simulink model "VehicleModel"  (R2020b)
settings: Solver=FixedStepAuto  StartTime=0.0  StopTime=1068  FixedStep=0.1  RelTol=1e-3
model workspace (MAT data in the model file):
  t : mpt.Parameter (value not decoded)
(part 4 of 5)

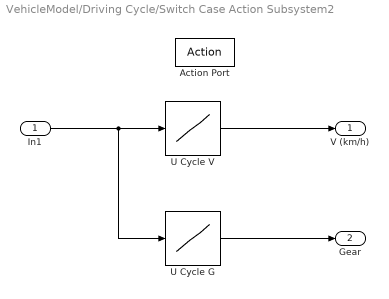
== system VehicleModel/Driving Cycle/Switch Case Action Subsystem2 ==
  In1 : Inport
  Action Port : ActionPort  ActionPortLabel=case [ 2 ]:
  " U Cycle V" : Lookup_n-D  NumberOfTableDimensions=1  BreakpointsForDimension1=|  Table=|  InternalRulePriority=Speed  RndMeth=Simplest  InputSameDT=on
      | [0
      | 1
      | 2
      | 3
      | 4
      | 5
      | 6
      | 7
      | 8
      | 9
      | 10
      | 11
      | 12
      | 13
      | 14
      | 15
      | 16
      | 17
      | 18
      | 19
      | 20
      | 21
      | 22
      | 23
      | 24
      | 25
      | 26
      | 27
      | 28
      | 29
      | 30
      | 31
      | 32
      | 33
      | 34
      | 35
      | 36
      | 37
      | 38
      | 39
      | 40
      | 41
      | 42
      | 43
      | 44
      | 45
      | 46
      | 47
      | 48
      | 49
      | 50
      | 51
      | 52
      | 53
      | 54
      | 55
      | 56
      | 57
      | 58
      | 59
      | 60
      | 61
      | 62
      | 63
      | 64
      | 65
      | 66
      | 67
      | 68
      | 69
      | 70
      | 71
      | 72
      | 73
      | 74
      | 75
      | 76
      | 77
      | 78
      | 79
      | 80
      | 81
      | 82
      | 83
      | 84
      | 85
      | 86
      | 87
      | 88
      | 89
      | 90
      | 91
      | 92
      | 93
      | 94
      | 95
      | 96
      | 97
      | 98
      | 99
      | 100
      | 101
      | 102
      | 103
      | 104
      | 105
      | 106
      | 107
      | 108
      | 109
      | 110
      | 111
      | 112
      | 113
      | 114
      | 115
      | 116
      | 117
      | 118
      | 119
      | 120
      | 121
      | 122
      | 123
      | 124
      | 125
      | 126
      | 127
      | 128
      | 129
      | 130
      | 131
      | 132
      | 133
      | 134
      | 135
      | 136
      | 137
      | 138
      | 139
      | 140
      | 141
      | 142
      | 143
      | 144
      | 145
      | 146
      | 147
      | 148
      | 149
      | 150
      | 151
      | 152
      | 153
      | 154
      | 155
      | 156
      | 157
      | 158
      | 159
      | 160
      | 161
      | 162
      | 163
      | 164
      | 165
      | 166
      | 167
      | 168
      | 169
      | 170
      | 171
      | 172
      | 173
      | 174
      | 175
      | 176
      | 177
      | 178
      | 179
      | 180
      | 181
      | 182
      | 183
      | 184
      | 185
      | 186
      | 187
      | 188
      | 189
      | 190
      | 191
      | 192
      | 193
      | 194
      | 195
      | 196
      | 197
      | 198
      | 199
      | 200
      | 201
      | 202
      | 203
      | 204
      | 205
      | 206
      | 207
      | 208
      | 209
      | 210
      | 211
      | 212
      | 213
      | 214
      | 215
      | 216
      | 217
      | 218
      | 219
      | 220
      | 221
      | 222
      | 223
      | 224
      | 225
      | 226
      | 227
      | 228
      | 229
      | 230
      | 231
      | 232
      | 233
      | 234
      | 235
      | 236
      | 237
      | 238
      | 239
      | 240
      | 241
      | 242
      | 243
      | 244
      | 245
      | 246
      | 247
      | 248
      | 249
      | 250
      | 251
      | 252
      | 253
      | 254
      | 255
      | 256
      | 257
      | 258
      | 259
      | 260
      | 261
      | 262
      | 263
      | 264
      | 265
      | 266
      | 267
      | 268
      | 269
      | 270
      | 271
      | 272
      | 273
      | 274
      | 275
      | 276
      | 277
      | 278
      | 279
      | 280
      | 281
      | 282
      | 283
      | 284
      | 285
      | 286
      | 287
      | 288
      | 289
      | 290
      | 291
      | 292
      | 293
      | 294
      | 295
      | 296
      | 297
      | 298
      | 299
      | 300
      | 301
      | 302
      | 303
      | 304
      | 305
      | 306
      | 307
      | 308
      | 309
      | 310
      | 311
      | 312
      | 313
      | 314
      | 315
      | 316
      | 317
      | 318
      | 319
      | 320
      | 321
      | 322
      | 323
      | 324
      | 325
      | 326
      | 327
      | 328
      | 329
      | 330
      | 331
      | 332
      | 333
      | 334
      | 335
      | 336
      | 337
      | 338
      | 339
      | 340
      | 341
      | 342
      | 343
      | 344
      | 345
      | 346
      | 347
      | 348
      | 349
      | 350
      | 351
      | 352
      | 353
      | 354
      | 355
      | 356
      | 357
      | 358
      | 359
      | 360
      | 361
      | 362
      | 363
      | 364
      | 365
      | 366
      | 367
      | 368
      | 369
      | 370
      | 371
      | 372
      | 373
      | 374
      | 375
      | 376
      | 377
      | 378
      | 379
      | 380
      | 381
      | 382
      | 383
      | 384
      | 385
      | 386
      | 387
      | 388
      | 389
      | 390
      | 391
      | 392
      | 393
      | 394
      | 395
      | 396
      | 397
      | 398
      | 399
      | 400
      | 401
      | 402
      | 403
      | 404
      | 405
      | 406
      | 407
      | 408
      | 409
      | 410
      | 411
      | 412
      | 413
      | 414
      | 415
      | 416
      | 417
      | 418
      | 419
      | 420
      | 421
      | 422
      | 423
      | 424
      | 425
      | 426
      | 427
      | 428
      | 429
      | 430
      | 431
      | 432
      | 433
      | 434
      | 435
      | 436
      | 437
      | 438
      | 439
      | 440
      | 441
      | 442
      | 443
      | 444
      | 445
      | 446
      | 447
      | 448
      | 449
      | 450
      | 451
      | 452
      | 453
      | 454
      | 455
      | 456
      | 457
      | 458
      | 459
      | 460
      | 461
      | 462
      | 463
      | 464
      | 465
      | 466
      | 467
      | 468
      | 469
      | 470
      | 471
      | 472
      | 473
      | 474
      | 475
      | 476
      | 477
      | 478
      | 479
      | 480
      | 481
      | 482
      | 483
      | 484
      | 485
      | 486
      | 487
      | 488
      | 489
      | 490
      | 491
      | 492
      | 493
      | 494
      | 495
      | 496
      | 497
      | 498
      | 499
      | 500
      | 501
      | 502
      | 503
      | 504
      | 505
      | 506
      | 507
      | 508
      | 509
      | 510
      | 511
      | 512
      | 513
      | 514
      | 515
      | 516
      | 517
      | 518
      | 519
      | 520
      | 521
      | 522
      | 523
      | 524
      | 525
      | 526
      | 527
      | 528
      | 529
      | 530
      | 531
      | 532
      | 533
      | 534
      | 535
      | 536
      | 537
      | 538
      | 539
      | 540
      | 541
      | 542
      | 543
      | 544
      | 545
      | 546
      | 547
      | 548
      | 549
      | 550
      | 551
      | 552
      | 553
      | 554
      | 555
      | 556
      | 557
      | 558
      | 559
      | 560
      | 561
      | 562
      | 563
      | 564
      | 565
      | 566
      | 567
      | 568
      | 569
      | 570
      | 571
      | 572
      | 573
      | 574
      | 575
      | 576
      | 577
      | 578
      | 579
      | 580
      | 581
      | 582
      | 583
      | 584
      | 585
      | 586
      | 587
      | 588
      | 589
      | 590
      | 591
      | 592
      | 593
      | 594
      | 595
      | 596
      | 597
      | 598
      | 599
      | 600
      | 601
      | 602
      | 603
      | 604
      | 605
      | 606
      | 607
      | 608
      | 609
      | 610
      | 611
      | 612
      | 613
      | 614
      | 615
      | 616
      | 617
      | 618
      | 619
      | 620
      | 621
      | 622
      | 623
      | 624
      | 625
      | 626
      | 627
      | 628
      | 629
      | 630
      | 631
      | 632
      | 633
      | 634
      | 635
      | 636
      | 637
      | 638
      | 639
      | 640
      | 641
      | 642
      | 643
      | 644
      | 645
      | 646
      | 647
      | 648
      | 649
      | 650
      | 651
      | 652
      | 653
      | 654
      | 655
      | 656
      | 657
      | 658
      | 659
      | 660
      | 661
      | 662
      | 663
      | 664
      | 665
      | 666
      | 667
      | 668
      | 669
      | 670
      | 671
      | 672
      | 673
      | 674
      | 675
      | 676
      | 677
      | 678
      | 679
      | 680
      | 681
      | 682
      | 683
      | 684
      | 685
      | 686
      | 687
      | 688
      | 689
      | 690
      | 691
      | 692
      | 693
      | 694
      | 695
      | 696
      | 697
      | 698
      | 699
      | 700
      | 701
      | 702
      | 703
      | 704
      | 705
      | 706
      | 707
      | 708
      | 709
      | 710
      | 711
      | 712
      | 713
      | 714
      | 715
      | 716
      | 717
      | 718
      | 719
      | 720
      | 721
      | 722
      | 723
      | 724
      | 725
      | 726
      | 727
      | 728
      | 729
      | 730
      | 731
      | 732
      | 733
      | 734
      | 735
      | 736
      | 737
      | 738
      | 739
      | 740
      | 741
      | 742
      | 743
      | 744
      | 745
      | 746
      | 747
      | 748
      | 749
      | 750
      | 751
      | 752
      | 753
      | 754
      | 755
      | 756
      | 757
      | 758
      | 759
      | 760
      | 761
      | 762
      | 763
      | 764
      | 765
      | 766
      | 767
      | 768
      | 769
      | 770
      | 771
      | 772
      | 773
      | 774
      | 775
      | 776
      | 777
      | 778
      | 779
      | 780
      | 781
      | 782
      | 783
      | 784
      | 785
      | 786
      | 787
      | 788
      | 789
      | 790
      | 791
      | 792
      | 793
      | 794
      | 795
      | 796
      | 797
      | 798
      | 799
      | 800
      | 801
      | 802
      | 803
      | 804
      | 805
      | 806
      | 807
      | 808
      | 809
      | 810
      | 811
      | 812
      | 813
      | 814
      | 815
      | 816
      | 817
      | 818
      | 819
      | 820
      | 821
      | 822
      | 823
      | 824
      | 825
      | 826
      | 827
      | 828
      | 829
      | 830
      | 831
      | 832
      | 833
      | 834
      | 835
      | 836
      | 837
      | 838
      | 839
      | 840
      | 841
      | 842
      | 843
      | 844
      | 845
      | 846
      | 847
      | 848
      | 849
      | 850
      | 851
      | 852
      | 853
      | 854
      | 855
      | 856
      | 857
      | 858
      | 859
      | 860
      | 861
      | 862
      | 863
      | 864
      | 865
      | 866
      | 867
      | 868
      | 869
      | 870
      | 871
      | 872
      | 873
      | 874
      | 875
      | 876
      | 877
      | 878
      | 879
      | 880
      | 881
      | 882
      | 883
      | 884
      | 885
      | 886
      | 887
      | 888
      | 889
      | 890
      | 891
      | 892
      | 893
      | 894
      | 895
      | 896
      | 897
      | 898
      | 899
      | 900
      | 901
      | 902
      | 903
      | 904
      | 905
      | 906
      | 907
      | 908
      | 909
      | 910
      | 911
      | 912
      | 913
      | 914
      | 915
      | 916
      | 917
      | 918
      | 919
      | 920
      | 921
      | 922
      | 923
      | 924
      | 925
      | 926
      | 927
      | 928
      | 929
      | 930
      | 931
      | 932
      | 933
      | 934
      | 935
      | 936
      | 937
      | 938
      | 939
      | 940
      | 941
      | 942
      | 943
      | 944
      | 945
      | 946
      | 947
      | 948
      | 949
      | 950
      | 951
      | 952
      | 953
      | 954
      | 955
      | 956
      | 957
      | 958
      | 959
      | 960
      | 961
      | 962
      | 963
      | 964
      | 965
      | 966
      | 967
      | 968
      | 969
      | 970
      | 971
      | 972
      | 973
      | 974
      | 975
      | 976
      | 977
      | 978
      | 979
      | 980
      | 981
      | 982
      | 983
      | 984
      | 985
      | 986
      | 987
      | 988
      | 989
      | 990
      | 991
      | 992
      | 993]
      | [0
      | 0
      | 0
      | 0
      | 0
      | 0
      | 0
      | 0
      | 0
      | 0
      | 0
      | 0
      | 0
      | 0
      | 0
      | 0
      | 0
      | 0
      | 0
      | 0
      | 0
      | 0.700000000000000
      | 2.10000000000000
      | 9.20000000000000
      | 15.6000000000000
      | 19.8000000000000
      | 19.8000000000000
      | 22.7000000000000
      | 25.5000000000000
      | 29.8000000000000
      | 34
      | 36.9000000000000
      | 38.3000000000000
      | 40.4000000000000
      | 43.2000000000000
      | 46.1000000000000
      | 46.1000000000000
      | 46.1000000000000
      | 44.6000000000000
      | 46.1000000000000
      | 48.2000000000000
      | 48.9000000000000
      | 48.2000000000000
      | 46.8000000000000
      | 44.6000000000000
      | 42.5000000000000
      | 41.8000000000000
      | 41.1000000000000
      | 39.7000000000000
      | 36.1000000000000
      | 34.7000000000000
      | 34.7000000000000
      | 36.9000000000000
      | 36.1000000000000
      | 36.1000000000000
      | 34.7000000000000
      | 32.6000000000000
      | 29.1000000000000
      | 24.1000000000000
      | 20.6000000000000
      | 15.6000000000000
      | 11.3000000000000
      | 9.20000000000000
      | 9.20000000000000
      | 9.20000000000000
      | 9.90000000000000
      | 10.6000000000000
      | 12
      | 11.3000000000000
      | 7.80000000000000
      | 1.40000000000000
      | 0
      | 0
      | 0
      | 0
      | 0
      | 0
      | 0
      | 0
      | 0
      | 0
      | 0
      | 0
      | 0
      | 0
      | 0
      | 0
      | 0
      | 0
      | 0
      | 0
      | 0
      | 0
      | 0.700000000000000
      | 2.10000000000000
      | 9.20000000000000
      | 15.6000000000000
      | 19.8000000000000
      | 19.8000000000000
      | 22.7000000000000
      | 25.5000000000000
      | 29.8000000000000
      | 34
      | 36.9000000000000
      | 38.3000000000000
      | 40.4000000000000
      | 43.2000000000000
      | 46.1000000000000
      | 46.1000000000000
      | 46.1000000000000
      | 44.6000000000000
      | 46.1000000000000
      | 48.2000000000000
      | 48.9000000000000
      | 48.2000000000000
      | 46.8000000000000
      | 44.6000000000000
      | 42.5000000000000
      | 41.8000000000000
      | 41.1000000000000
      | 39.7000000000000
      | 36.1000000000000
      | 34.7000000000000
      | 34.7000000000000
      | 36.9000000000000
      | 36.1000000000000
      | 36.1000000000000
      | 34.7000000000000
      | 32.6000000000000
      | 29.1000000000000
      | 24.1000000000000
      | 20.6000000000000
      | 15.6000000000000
      | 11.3000000000000
      | 9.20000000000000
      | 9.20000000000000
      | 9.20000000000000
      | 9.90000000000000
      | 10.6000000000000
      | 12
      | 11.3000000000000
      | 7.80000000000000
      | 1.40000000000000
      | 0
      | 0
      | 0
      | 0
      | 0
      | 0
      | 0
      | 0
      | 0
      | 0
      | 0.700000000000000
      | 1.50000000000000
      | 4.40000000000000
      | 5.90000000000000
      | 7.30000000000000
      | 9.50000000000000
      | 8.10000000000000
      | 3.70000000000000
      | 2.90000000000000
      | 4.40000000000000
      | 0.700000000000000
      | 0
      | 0
      | 2.20000000000000
      | 2.20000000000000
      | 2.90000000000000
      | 7.30000000000000
      | 5.90000000000000
      | 7.30000000000000
      | 8.80000000000000
      | 11
      | 15.4000000000000
      | 13.9000000000000
      | 11.7000000000000
      | 11
      | 5.10000000000000
      | 0
      | 0
      | 0
      | 0
      | 0
      | 0
      | 0
      | 0
      | 0
      | 0
      | 0
      | 0
      | 0
      | 0
      | 0
      | 0
      | 0
      | 0
      | 0
      | 0
      | 0
      | 0
      | 0
      | 0
      | 0
      | 0
      | 0
      | 0
      | 0
      | 0.700000000000000
      | 11
      | 13.2000000000000
      | 13.9000000000000
      | 14.7000000000000
      | 15.4000000000000
      | 16.9000000000000
      | 16.1000000000000
      | 15.4000000000000
      | 13.9000000000000
      | 13.2000000000000
      | 13.2000000000000
      | 15.4000000000000
      | 16.9000000000000
      | 16.1000000000000
      | 14.7000000000000
      | 13.2000000000000
      | 13.9000000000000
      | 14.7000000000000
      | 18.3000000000000
      | 22
      | 30.1000000000000
      | 32.3000000000000
      | 32.3000000000000
      | 38.1000000000000
      | 38.1000000000000
      | 38.1000000000000
      | 38.1000000000000
      | 38.9000000000000
      | 39.6000000000000
      | 40.3000000000000
      | 40.3000000000000
      | 41.1000000000000
      | 43.3000000000000
      | 44.7000000000000
      | 45.5000000000000
      | 44
      | 44
      | 43.3000000000000
      | 41.8000000000000
      | 38.9000000000000
      | 34.5000000000000
      | 33
      | 33.7000000000000
      | 36.7000000000000
      | 37.4000000000000
      | 40.3000000000000
      | 41.1000000000000
      | 41.1000000000000
      | 38.9000000000000
      | 37.4000000000000
      | 35.9000000000000
      | 34.5000000000000
      | 32.3000000000000
      | 30.8000000000000
      | 27.9000000000000
      | 26.4000000000000
      | 24.2000000000000
      | 23.5000000000000
      | 22.7000000000000
      | 21.3000000000000
      | 19.1000000000000
      | 16.9000000000000
      | 11
      | 6.60000000000000
      | 5.10000000000000
      | 4.40000000000000
      | 2.20000000000000
      | 0
      | 0
      | 0
      | 2.20000000000000
      | 5.10000000000000
      | 13.9000000000000
      | 22.7000000000000
      | 27.1000000000000
      | 27.1000000000000
      | 22.7000000000000
      | 18.3000000000000
      | 11.7000000000000
      | 8.80000000000000
      | 6.60000000000000
      | 3.70000000000000
      | 2.90000000000000
      | 4.40000000000000
      | 11
      | 11.7000000000000
      | 11.7000000000000
      | 11
      | 8.80000000000000
      | 6.60000000000000
      | 7.30000000000000
      | 5.90000000000000
      | 4.40000000000000
      | 2.20000000000000
      | 0.700000000000000
      | 0
      | 0
      | 0
      | 0
      | 0
      | 0
      | 0
      | 2
      | 6.90000000000000
      | 10.8000000000000
      | 12.3000000000000
      | 14.3000000000000
      | 19.7000000000000
      | 21.2000000000000
      | 23.7000000000000
      | 28.1000000000000
      | 31
      | 31.5000000000000
      | 33
      | 34
      | 31
      | 24.1000000000000
      | 15.8000000000000
      | 10.8000000000000
      | 6.40000000000000
      | 2.50000000000000
      | 1.50000000000000
      | 0
      | 0
      | 0.500000000000000
      | 6.40000000000000
      | 13.8000000000000
      | 19.2000000000000
      | 19.2000000000000
      | 21.2000000000000
      | 22.7000000000000
      | 25.1000000000000
      | 28.6000000000000
      | 33.5000000000000
      | 37
      | 37.9000000000000
      | 40.9000000000000
      | 44.4000000000000
      | 47.3000000000000
      | 50.8000000000000
      | 52.2000000000000
      | 51.3000000000000
      | 48.8000000000000
      | 48.8000000000000
      | 50.8000000000000
      | 50.8000000000000
      | 47.3000000000000
      | 40.4000000000000
      | 29.1000000000000
      | 23.7000000000000
      | 25.1000000000000
      | 27.1000000000000
      | 29.1000000000000
      | 33.5000000000000
      | 36.5000000000000
      | 38.9000000000000
      | 41.9000000000000
      | 44.8000000000000
      | 47.8000000000000
      | 50.8000000000000
      | 53.2000000000000
      | 54.7000000000000
      | 54.2000000000000
      | 54.7000000000000
      | 55.2000000000000
      | 56.7000000000000
      | 57.2000000000000
      | 57.2000000000000
      | 57.7000000000000
      | 57.2000000000000
      | 57.2000000000000
      | 56.7000000000000
      | 56.7000000000000
      | 56.2000000000000
      | 54.7000000000000
      | 54.7000000000000
      | 52.2000000000000
      | 48.8000000000000
      | 43.9000000000000
      | 43.4000000000000
      | 44.4000000000000
      | 43.4000000000000
      | 38.4000000000000
      | 34.5000000000000
      | 33.5000000000000
      | 34
      | 37.5000000000000
      | 41.9000000000000
      | 45.8000000000000
      | 49.3000000000000
      | 48.3000000000000
      | 46.3000000000000
      | 43.4000000000000
      | 38.9000000000000
      | 33.5000000000000
      | 32
      | 33
      | 34
      | 34
      | 33.5000000000000
      | 33
      | 33
      | 33
      | 33.5000000000000
      | 35
      | 35.5000000000000
      | 36
      | 37
      | 37
      | 37.5000000000000
      | 37.5000000000000
      | 38.4000000000000
      | 38.9000000000000
      | 38.4000000000000
      | 38.4000000000000
      | 40.4000000000000
      | 42.4000000000000
      | 42.9000000000000
      | 42.4000000000000
      | 41.4000000000000
      | 38.9000000000000
      | 30.6000000000000
      | 19.7000000000000
      | 13.8000000000000
      | 12.3000000000000
      | 10.8000000000000
      | 4.40000000000000
      | 0.500000000000000
      | 0
      | 0
      | 0
      | 0
      | 0
      | 0
      | 0
      | 0.700000000000000
      | 3.60000000000000
      | 5.80000000000000
      | 8.70000000000000
      | 15.9000000000000
      | 21
      | 26.7000000000000
      | 32.5000000000000
      | 34.7000000000000
      | 36.9000000000000
      | 39
      | 41.2000000000000
      | 43.4000000000000
      | 45.5000000000000
      | 47
      | 48.4000000000000
      | 48.4000000000000
      | 48.4000000000000
      | 47.7000000000000
      | 47.7000000000000
      | 47
      | 47.7000000000000
      | 48.4000000000000
      | 49.2000000000000
      | 49.2000000000000
      | 49.2000000000000
      | 49.2000000000000
      | 44.1000000000000
      | 36.1000000000000
      | 34
      | 31.1000000000000
      | 30.4000000000000
      | 31.8000000000000
      | 32.5000000000000
      | 33.3000000000000
      | 31.8000000000000
      | 31.1000000000000
      | 28.9000000000000
      | 18.1000000000000
      | 15.9000000000000
      | 18.1000000000000
      | 23.1000000000000
      | 27.5000000000000
      | 33.3000000000000
      | 36.9000000000000
      | 41.2000000000000
      | 44.1000000000000
      | 46.3000000000000
      | 46.3000000000000
      | 46.3000000000000
      | 44.1000000000000
      | 41.2000000000000
      | 35.4000000000000
      | 26.7000000000000
      | 15.9000000000000
      | 6.50000000000000
      | 3.60000000000000
      | 0.700000000000000
      | 0
      | 0
      | 0
      | 0
      | 0
      | 0
      | 0
      | 0
      | 0
      | 0
      | 0
      | 0
      | 0
      | 0
      | 0
      | 0
      | 0
      | 0
      | 0
      | 0
      | 0
      | 0
      | 0
      | 0
      | 0
      | 0
      | 0
      | 0
      | 0
      | 2
      | 8.50000000000000
      | 13.4000000000000
      | 14.9000000000000
      | 20.4000000000000
      | 27.3000000000000
      | 33.8000000000000
      | 39.8000000000000
      | 44.7000000000000
      | 45.2000000000000
      | 46.2000000000000
      | 42.3000000000000
      | 38.8000000000000
      | 39.3000000000000
      | 43.3000000000000
      | 46.2000000000000
      | 46.2000000000000
      | 43.3000000000000
      | 38.3000000000000
      | 29.3000000000000
      | 25.9000000000000
      | 26.4000000000000
      | 31.3000000000000
      | 36.8000000000000
      | 41.3000000000000
      | 42.8000000000000
      | 41.8000000000000
      | 38.8000000000000
      | 33.3000000000000
      | 25.4000000000000
      | 18.4000000000000
      | 14.4000000000000
      | 6.50000000000000
      | 0.500000000000000
      | 0
      | 0
      | 0
      | 0
      | 0
      | 0
      | 0
      | 0
      | 0
      | 0
      | 0
      | 0
      | 0
      | 5.30000000000000
      | 9.20000000000000
      | 11
      | 12.7000000000000
      | 11.8000000000000
      | 8.80000000000000
      | 7.50000000000000
      | 7.90000000000000
      | 8.30000000000000
      | 9.20000000000000
      | 10.5000000000000
      | 9.60000000000000
      | 8.80000000000000
      | 8.80000000000000
      | 6.60000000000000
      | 2.60000000000000
      | 0.400000000000000
      | 0
      | 0
      | 0
      | 0
      | 0
      | 0
      | 0
      | 0
      | 0
      | 0
      | 0
      | 0
      | 0
      | 0
      | 0
      | 0
      | 0
      | 0
      | 0
      | 0
      | 0
      | 0
      | 0
      | 0
      | 0
      | 0
      | 3.10000000000000
      | 7.90000000000000
      | 13.2000000000000
      | 13.2000000000000
      | 7.50000000000000
      | 3.50000000000000
      | 1.30000000000000
      | 0
      | 0
      | 0
      | 0
      | 1.80000000000000
      | 9.60000000000000
      | 17.1000000000000
      | 21.5000000000000
      | 24.1000000000000
      | 25.4000000000000
      | 22.8000000000000
      | 18.4000000000000
      | 12.3000000000000
      | 6.60000000000000
      | 1.30000000000000
      | 0
      | 0
      | 0
      | 0
      | 0
      | 0
      | 0
      | 0
      | 0
      | 0
      | 0
      | 0
      | 0
      | 0
      | 0
      | 0
      | 0
      | 0
      | 0
      | 0
      | 0
      | 0
      | 0
      | 0
      | 0
      | 0
      | 0
      | 0
      | 0
      | 0
      | 0
      | 0
      | 0
      | 0
      | 0
      | 0
      | 0
      | 0
      | 0
      | 0
      | 0
      | 0
      | 0
      | 0
      | 0
      | 0
      | 0
      | 0
      | 0
      | 0
      | 0
      | 0
      | 0
      | 0
      | 0
      | 0
      | 0
      | 0
      | 0
      | 0
      | 0
      | 0
      | 0.400000000000000
      | 4.40000000000000
      | 9.60000000000000
      | 16.7000000000000
      | 18.4000000000000
      | 20.2000000000000
      | 23.2000000000000
      | 26.7000000000000
      | 30.7000000000000
      | 31.6000000000000
      | 32
      | 34.2000000000000
      | 36
      | 38.1000000000000
      | 39.9000000000000
      | 41.7000000000000
      | 42.1000000000000
      | 40.8000000000000
      | 39
      | 34.2000000000000
      | 27.6000000000000
      | 20.6000000000000
      | 16.7000000000000
      | 14.5000000000000
      | 14
      | 14
      | 14.5000000000000
      | 13.2000000000000
      | 11
      | 9.20000000000000
      | 7.50000000000000
      | 3.50000000000000
      | 1.30000000000000
      | 0
      | 0
      | 0
      | 0
      | 0
      | 0
      | 0
      | 0
      | 0
      | 0
      | 0
      | 0
      | 0
      | 0
      | 0
      | 0
      | 0
      | 0
      | 3.80000000000000
      | 3.10000000000000
      | 3.10000000000000
      | 4.60000000000000
      | 6.10000000000000
      | 4.60000000000000
      | 0.800000000000000
      | 3.80000000000000
      | 11.5000000000000
      | 15.3000000000000
      | 10.7000000000000
      | 6.90000000000000
      | 6.10000000000000
      | 8.40000000000000
      | 13
      | 17.6000000000000
      | 22.2000000000000
      | 25.3000000000000
      | 28.3000000000000
      | 31.4000000000000
      | 32.2000000000000
      | 32.2000000000000
      | 29.9000000000000
      | 24.5000000000000
      | 19.1000000000000
      | 14.6000000000000
      | 7.70000000000000
      | 1.50000000000000
      | 2.30000000000000
      | 6.10000000000000
      | 10
      | 10
      | 11.5000000000000
      | 13.8000000000000
      | 19.9000000000000
      | 23
      | 26.8000000000000
      | 32.9000000000000
      | 36.8000000000000
      | 38.3000000000000
      | 38.3000000000000
      | 39.8000000000000
      | 38.3000000000000
      | 34.5000000000000
      | 30.6000000000000
      | 24.5000000000000
      | 19.9000000000000
      | 19.9000000000000
      | 22.2000000000000
      | 25.3000000000000
      | 29.9000000000000
      | 32.9000000000000
      | 33.7000000000000
      | 32.9000000000000
      | 29.9000000000000
      | 29.1000000000000
      | 27.6000000000000
      | 26
      | 24.5000000000000
      | 24.5000000000000
      | 22.2000000000000
      | 18.4000000000000
      | 16.9000000000000
      | 15.3000000000000
      | 14.6000000000000
      | 11.5000000000000
      | 6.90000000000000
      | 0.800000000000000
      | 0
      | 0
      | 0
      | 0
      | 0
      | 0
      | 0
      | 4.60000000000000
      | 10.7000000000000
      | 13
      | 14.6000000000000
      | 16.1000000000000
      | 16.1000000000000
      | 14.6000000000000
      | 12.3000000000000
      | 7.70000000000000
      | 5.40000000000000
      | 6.10000000000000
      | 6.90000000000000
      | 3.80000000000000
      | 3.80000000000000
      | 4.60000000000000
      | 4.60000000000000
      | 1.50000000000000
      | 0
      | 1.50000000000000
      | 2.30000000000000
      | 3.10000000000000
      | 2.30000000000000
      | 1.50000000000000
      | 0
      | 0
      | 0.800000000000000
      | 2.30000000000000
      | 3.10000000000000
      | 3.80000000000000
      | 4.60000000000000
      | 3.10000000000000
      | 0
      | 0.800000000000000
      | 3.10000000000000
      | 4.60000000000000
      | 4.60000000000000
      | 3.80000000000000
      | 3.10000000000000
      | 0.800000000000000
      | 0
      | 3.10000000000000
      | 2.30000000000000
      | 0
      | 0
      | 0
      | 0
      | 0
      | 0
      | 0
      | 0
      | 0.700000000000000
      | 6.40000000000000
      | 12.1000000000000
      | 16.3000000000000
      | 18.5000000000000
      | 20.6000000000000
      | 22
      | 22.7000000000000
      | 24.9000000000000
      | 26.3000000000000
      | 27.7000000000000
      | 28.4000000000000
      | 31.2000000000000
      | 32.7000000000000
      | 34.8000000000000
      | 35.5000000000000
      | 35.5000000000000
      | 34.8000000000000
      | 33.4000000000000
      | 32
      | 30.5000000000000
      | 28.4000000000000
      | 27.7000000000000
      | 27
      | 25.6000000000000
      | 24.1000000000000
      | 19.9000000000000
      | 12.8000000000000
      | 5.70000000000000
      | 7.80000000000000
      | 12.8000000000000
      | 17.8000000000000
      | 19.9000000000000
      | 18.5000000000000
      | 17
      | 16.3000000000000
      | 17.8000000000000
      | 19.2000000000000
      | 19.9000000000000
      | 21.3000000000000
      | 18.5000000000000
      | 17.8000000000000
      | 16.3000000000000
      | 18.5000000000000
      | 19.2000000000000
      | 17.8000000000000
      | 12.8000000000000
      | 5.70000000000000
      | 0
      | 0
      | 3.60000000000000
      | 10.7000000000000
      | 19.2000000000000
      | 26.3000000000000
      | 31.2000000000000
      | 35.5000000000000
      | 39.1000000000000
      | 41.9000000000000
      | 42.6000000000000
      | 44
      | 42.6000000000000
      | 41.2000000000000
      | 39.1000000000000
      | 36.9000000000000
      | 31.2000000000000
      | 27
      | 18.5000000000000
      | 11.4000000000000
      | 11.4000000000000
      | 15.6000000000000
      | 22
      | 24.9000000000000
      | 27
      | 29.1000000000000
      | 30.5000000000000
      | 32
      | 32
      | 31.2000000000000
      | 32.7000000000000
      | 32
      | 32
      | 31.2000000000000
      | 29.8000000000000
      | 28.4000000000000
      | 23.4000000000000
      | 21.3000000000000
      | 20.6000000000000
      | 22.7000000000000
      | 22
      | 22
      | 23.4000000000000
      | 26.3000000000000
      | 28.4000000000000
      | 29.8000000000000
      | 29.8000000000000
      | 30.5000000000000
      | 29.1000000000000
      | 29.1000000000000
      | 27.7000000000000
      | 26.3000000000000
      | 24.9000000000000
      | 22.7000000000000
      | 21.3000000000000
      | 17
      | 11.4000000000000
      | 5.70000000000000
      | 0.700000000000000
      | 0
      | 0
      | 0
      | 0
      | 0
      | 0]
  U Cycle G : Lookup_n-D  NumberOfTableDimensions=1  BreakpointsForDimension1=|  Table=|  InternalRulePriority=Speed  RndMeth=Simplest  InputSameDT=on
      | [0
      | 1
      | 2
      | 3
      | 4
      | 5
      | 6
      | 7
      | 8
      | 9
      | 10
      | 11
      | 12
      | 13
      | 14
      | 15
      | 16
      | 17
      | 18
      | 19
      | 20
      | 21
      | 22
      | 23
      | 24
      | 25
      | 26
      | 27
      | 28
      | 29
      | 30
      | 31
      | 32
      | 33
      | 34
      | 35
      | 36
      | 37
      | 38
      | 39
      | 40
      | 41
      | 42
      | 43
      | 44
      | 45
      | 46
      | 47
      | 48
      | 49
      | 50
      | 51
      | 52
      | 53
      | 54
      | 55
      | 56
      | 57
      | 58
      | 59
      | 60
      | 61
      | 62
      | 63
      | 64
      | 65
      | 66
      | 67
      | 68
      | 69
      | 70
      | 71
      | 72
      | 73
      | 74
      | 75
      | 76
      | 77
      | 78
      | 79
      | 80
      | 81
      | 82
      | 83
      | 84
      | 85
      | 86
      | 87
      | 88
      | 89
      | 90
      | 91
      | 92
      | 93
      | 94
      | 95
      | 96
      | 97
      | 98
      | 99
      | 100
      | 101
      | 102
      | 103
      | 104
      | 105
      | 106
      | 107
      | 108
      | 109
      | 110
      | 111
      | 112
      | 113
      | 114
      | 115
      | 116
      | 117
      | 118
      | 119
      | 120
      | 121
      | 122
      | 123
      | 124
      | 125
      | 126
      | 127
      | 128
      | 129
      | 130
      | 131
      | 132
      | 133
      | 134
      | 135
      | 136
      | 137
      | 138
      | 139
      | 140
      | 141
      | 142
      | 143
      | 144
      | 145
      | 146
      | 147
      | 148
      | 149
      | 150
      | 151
      | 152
      | 153
      | 154
      | 155
      | 156
      | 157
      | 158
      | 159
      | 160
      | 161
      | 162
      | 163
      | 164
      | 165
      | 166
      | 167
      | 168
      | 169
      | 170
      | 171
      | 172
      | 173
      | 174
      | 175
      | 176
      | 177
      | 178
      | 179
      | 180
      | 181
      | 182
      | 183
      | 184
      | 185
      | 186
      | 187
      | 188
      | 189
      | 190
      | 191
      | 192
      | 193
      | 194
      | 195
      | 196
      | 197
      | 198
      | 199
      | 200
      | 201
      | 202
      | 203
      | 204
      | 205
      | 206
      | 207
      | 208
      | 209
      | 210
      | 211
      | 212
      | 213
      | 214
      | 215
      | 216
      | 217
      | 218
      | 219
      | 220
      | 221
      | 222
      | 223
      | 224
      | 225
      | 226
      | 227
      | 228
      | 229
      | 230
      | 231
      | 232
      | 233
      | 234
      | 235
      | 236
      | 237
      | 238
      | 239
      | 240
      | 241
      | 242
      | 243
      | 244
      | 245
      | 246
      | 247
      | 248
      | 249
      | 250
      | 251
      | 252
      | 253
      | 254
      | 255
      | 256
      | 257
      | 258
      | 259
      | 260
      | 261
      | 262
      | 263
      | 264
      | 265
      | 266
      | 267
      | 268
      | 269
      | 270
      | 271
      | 272
      | 273
      | 274
      | 275
      | 276
      | 277
      | 278
      | 279
      | 280
      | 281
      | 282
      | 283
      | 284
      | 285
      | 286
      | 287
      | 288
      | 289
      | 290
      | 291
      | 292
      | 293
      | 294
      | 295
      | 296
      | 297
      | 298
      | 299
      | 300
      | 301
      | 302
      | 303
      | 304
      | 305
      | 306
      | 307
      | 308
      | 309
      | 310
      | 311
      | 312
      | 313
      | 314
      | 315
      | 316
      | 317
      | 318
      | 319
      | 320
      | 321
      | 322
      | 323
      | 324
      | 325
      | 326
      | 327
      | 328
      | 329
      | 330
      | 331
      | 332
      | 333
      | 334
      | 335
      | 336
      | 337
      | 338
      | 339
      | 340
      | 341
      | 342
      | 343
      | 344
      | 345
      | 346
      | 347
      | 348
      | 349
      | 350
      | 351
      | 352
      | 353
      | 354
      | 355
      | 356
      | 357
      | 358
      | 359
      | 360
      | 361
      | 362
      | 363
      | 364
      | 365
      | 366
      | 367
      | 368
      | 369
      | 370
      | 371
      | 372
      | 373
      | 374
      | 375
      | 376
      | 377
      | 378
      | 379
      | 380
      | 381
      | 382
      | 383
      | 384
      | 385
      | 386
      | 387
      | 388
      | 389
      | 390
      | 391
      | 392
      | 393
      | 394
      | 395
      | 396
      | 397
      | 398
      | 399
      | 400
      | 401
      | 402
      | 403
      | 404
      | 405
      | 406
      | 407
      | 408
      | 409
      | 410
      | 411
      | 412
      | 413
      | 414
      | 415
      | 416
      | 417
      | 418
      | 419
      | 420
      | 421
      | 422
      | 423
      | 424
      | 425
      | 426
      | 427
      | 428
      | 429
      | 430
      | 431
      | 432
      | 433
      | 434
      | 435
      | 436
      | 437
      | 438
      | 439
      | 440
      | 441
      | 442
      | 443
      | 444
      | 445
      | 446
      | 447
      | 448
      | 449
      | 450
      | 451
      | 452
      | 453
      | 454
      | 455
      | 456
      | 457
      | 458
      | 459
      | 460
      | 461
      | 462
      | 463
      | 464
      | 465
      | 466
      | 467
      | 468
      | 469
      | 470
      | 471
      | 472
      | 473
      | 474
      | 475
      | 476
      | 477
      | 478
      | 479
      | 480
      | 481
      | 482
      | 483
      | 484
      | 485
      | 486
      | 487
      | 488
      | 489
      | 490
      | 491
      | 492
      | 493
      | 494
      | 495
      | 496
      | 497
      | 498
      | 499
      | 500
      | 501
      | 502
      | 503
      | 504
      | 505
      | 506
      | 507
      | 508
      | 509
      | 510
      | 511
      | 512
      | 513
      | 514
      | 515
      | 516
      | 517
      | 518
      | 519
      | 520
      | 521
      | 522
      | 523
      | 524
      | 525
      | 526
      | 527
      | 528
      | 529
      | 530
      | 531
      | 532
      | 533
      | 534
      | 535
      | 536
      | 537
      | 538
      | 539
      | 540
      | 541
      | 542
      | 543
      | 544
      | 545
      | 546
      | 547
      | 548
      | 549
      | 550
      | 551
      | 552
      | 553
      | 554
      | 555
      | 556
      | 557
      | 558
      | 559
      | 560
      | 561
      | 562
      | 563
      | 564
      | 565
      | 566
      | 567
      | 568
      | 569
      | 570
      | 571
      | 572
      | 573
      | 574
      | 575
      | 576
      | 577
      | 578
      | 579
      | 580
      | 581
      | 582
      | 583
      | 584
      | 585
      | 586
      | 587
      | 588
      | 589
      | 590
      | 591
      | 592
      | 593
      | 594
      | 595
      | 596
      | 597
      | 598
      | 599
      | 600
      | 601
      | 602
      | 603
      | 604
      | 605
      | 606
      | 607
      | 608
      | 609
      | 610
      | 611
      | 612
      | 613
      | 614
      | 615
      | 616
      | 617
      | 618
      | 619
      | 620
      | 621
      | 622
      | 623
      | 624
      | 625
      | 626
      | 627
      | 628
      | 629
      | 630
      | 631
      | 632
      | 633
      | 634
      | 635
      | 636
      | 637
      | 638
      | 639
      | 640
      | 641
      | 642
      | 643
      | 644
      | 645
      | 646
      | 647
      | 648
      | 649
      | 650
      | 651
      | 652
      | 653
      | 654
      | 655
      | 656
      | 657
      | 658
      | 659
      | 660
      | 661
      | 662
      | 663
      | 664
      | 665
      | 666
      | 667
      | 668
      | 669
      | 670
      | 671
      | 672
      | 673
      | 674
      | 675
      | 676
      | 677
      | 678
      | 679
      | 680
      | 681
      | 682
      | 683
      | 684
      | 685
      | 686
      | 687
      | 688
      | 689
      | 690
      | 691
      | 692
      | 693
      | 694
      | 695
      | 696
      | 697
      | 698
      | 699
      | 700
      | 701
      | 702
      | 703
      | 704
      | 705
      | 706
      | 707
      | 708
      | 709
      | 710
      | 711
      | 712
      | 713
      | 714
      | 715
      | 716
      | 717
      | 718
      | 719
      | 720
      | 721
      | 722
      | 723
      | 724
      | 725
      | 726
      | 727
      | 728
      | 729
      | 730
      | 731
      | 732
      | 733
      | 734
      | 735
      | 736
      | 737
      | 738
      | 739
      | 740
      | 741
      | 742
      | 743
      | 744
      | 745
      | 746
      | 747
      | 748
      | 749
      | 750
      | 751
      | 752
      | 753
      | 754
      | 755
      | 756
      | 757
      | 758
      | 759
      | 760
      | 761
      | 762
      | 763
      | 764
      | 765
      | 766
      | 767
      | 768
      | 769
      | 770
      | 771
      | 772
      | 773
      | 774
      | 775
      | 776
      | 777
      | 778
      | 779
      | 780
      | 781
      | 782
      | 783
      | 784
      | 785
      | 786
      | 787
      | 788
      | 789
      | 790
      | 791
      | 792
      | 793
      | 794
      | 795
      | 796
      | 797
      | 798
      | 799
      | 800
      | 801
      | 802
      | 803
      | 804
      | 805
      | 806
      | 807
      | 808
      | 809
      | 810
      | 811
      | 812
      | 813
      | 814
      | 815
      | 816
      | 817
      | 818
      | 819
      | 820
      | 821
      | 822
      | 823
      | 824
      | 825
      | 826
      | 827
      | 828
      | 829
      | 830
      | 831
      | 832
      | 833
      | 834
      | 835
      | 836
      | 837
      | 838
      | 839
      | 840
      | 841
      | 842
      | 843
      | 844
      | 845
      | 846
      | 847
      | 848
      | 849
      | 850
      | 851
      | 852
      | 853
      | 854
      | 855
      | 856
      | 857
      | 858
      | 859
      | 860
      | 861
      | 862
      | 863
      | 864
      | 865
      | 866
      | 867
      | 868
      | 869
      | 870
      | 871
      | 872
      | 873
      | 874
      | 875
      | 876
      | 877
      | 878
      | 879
      | 880
      | 881
      | 882
      | 883
      | 884
      | 885
      | 886
      | 887
      | 888
      | 889
      | 890
      | 891
      | 892
      | 893
      | 894
      | 895
      | 896
      | 897
      | 898
      | 899
      | 900
      | 901
      | 902
      | 903
      | 904
      | 905
      | 906
      | 907
      | 908
      | 909
      | 910
      | 911
      | 912
      | 913
      | 914
      | 915
      | 916
      | 917
      | 918
      | 919
      | 920
      | 921
      | 922
      | 923
      | 924
      | 925
      | 926
      | 927
      | 928
      | 929
      | 930
      | 931
      | 932
      | 933
      | 934
      | 935
      | 936
      | 937
      | 938
      | 939
      | 940
      | 941
      | 942
      | 943
      | 944
      | 945
      | 946
      | 947
      | 948
      | 949
      | 950
      | 951
      | 952
      | 953
      | 954
      | 955
      | 956
      | 957
      | 958
      | 959
      | 960
      | 961
      | 962
      | 963
      | 964
      | 965
      | 966
      | 967
      | 968
      | 969
      | 970
      | 971
      | 972
      | 973
      | 974
      | 975
      | 976
      | 977
      | 978
      | 979
      | 980
      | 981
      | 982
      | 983
      | 984
      | 985
      | 986
      | 987
      | 988
      | 989
      | 990
      | 991
      | 992
      | 993]
      | [0
      | 0
      | 0
      | 0
      | 0
      | 0
      | 0
      | 0
      | 0
      | 0
      | 0
      | 0
      | 0
      | 0
      | 0
      | 0
      | 0
      | 0
      | 0
      | 0
      | 1
      | 1
      | 1
      | 1
      | 2
      | 2
      | 2
      | 2
      | 2
      | 2
      | 2
      | 2
      | 2
      | 2
      | 2
      | 3
      | 3
      | 3
      | 3
      | 3
      | 3
      | 3
      | 3
      | 3
      | 3
      | 3
      | 3
      | 3
      | 3
      | 3
      | 2
      | 2
      | 2
      | 2
      | 2
      | 2
      | 2
      | 2
      | 2
      | 2
      | 2
      | 1
      | 1
      | 1
      | 1
      | 1
      | 1
      | 0
      | 0
      | 0
      | 0
      | 0
      | 0
      | 0
      | 0
      | 0
      | 0
      | 0
      | 0
      | 0
      | 0
      | 0
      | 0
      | 0
      | 0
      | 0
      | 0
      | 0
      | 0
      | 0
      | 0
      | 0
      | 1
      | 1
      | 1
      | 1
      | 2
      | 2
      | 2
      | 2
      | 2
      | 2
      | 2
      | 2
      | 2
      | 2
      | 2
      | 3
      | 3
      | 3
      | 3
      | 3
      | 3
      | 3
      | 3
      | 3
      | 3
      | 3
      | 3
      | 3
      | 3
      | 3
      | 2
      | 2
      | 2
      | 2
      | 2
      | 2
      | 2
      | 2
      | 2
      | 2
      | 2
      | 1
      | 1
      | 1
      | 1
      | 1
      | 1
      | 0
      | 0
      | 0
      | 0
      | 0
      | 0
      | 0
      | 0
      | 0
      | 0
      | 0
      | 0
      | 0
      | 1
      | 1
      | 1
      | 1
      | 1
      | 1
      | 1
      | 1
      | 1
      | 1
      | 0
      | 0
      | 0
      | 1
      | 1
      | 1
      | 1
      | 1
      | 1
      | 1
      | 1
      | 1
      | 1
      | 1
      | 1
      | 1
      | 0
      | 0
      | 0
      | 0
      | 0
      | 0
      | 0
      | 0
      | 0
      | 0
      | 0
      | 0
      | 0
      | 0
      | 0
      | 0
      | 0
      | 0
      | 0
      | 0
      | 0
      | 0
      | 0
      | 0
      | 0
      | 0
      | 0
      | 0
      | 0
      | 1
      | 1
      | 1
      | 1
      | 1
      | 1
      | 1
      | 1
      | 1
      | 1
      | 1
      | 1
      | 1
      | 1
      | 1
      | 1
      | 1
      | 1
      | 1
      | 1
      | 1
      | 1
      | 2
      | 2
      | 2
      | 2
      | 2
      | 2
      | 2
      | 2
      | 2
      | 2
      | 2
      | 2
      | 2
      | 2
      | 3
      | 3
      | 3
      | 3
      | 3
      | 3
      | 3
      | 3
      | 3
      | 3
      | 3
      | 3
      | 3
      | 3
      | 3
      | 3
      | 3
      | 3
      | 3
      | 3
      | 3
      | 2
      | 2
      | 2
      | 2
      | 0
      | 0
      | 0
      | 0
      | 0
      | 0
      | 0
      | 0
      | 0
      | 0
      | 1
      | 1
      | 1
      | 1
      | 1
      | 1
      | 2
      | 2
      | 2
      | 0
      | 0
      | 0
      | 1
      | 1
      | 1
      | 1
      | 1
      | 1
      | 1
      | 1
      | 1
      | 1
      | 1
      | 1
      | 0
      | 0
      | 0
      | 0
      | 0
      | 0
      | 0
      | 0
      | 1
      | 1
      | 1
      | 1
      | 1
      | 1
      | 1
      | 1
      | 1
      | 1
      | 2
      | 2
      | 2
      | 2
      | 0
      | 0
      | 0
      | 0
      | 0
      | 0
      | 0
      | 0
      | 1
      | 1
      | 1
      | 1
      | 1
      | 1
      | 1
      | 1
      | 1
      | 1
      | 2
      | 2
      | 2
      | 2
      | 2
      | 2
      | 3
      | 3
      | 3
      | 3
      | 3
      | 3
      | 3
      | 3
      | 3
      | 3
      | 2
      | 2
      | 2
      | 2
      | 2
      | 2
      | 2
      | 2
      | 2
      | 3
      | 3
      | 3
      | 4
      | 4
      | 4
      | 4
      | 4
      | 4
      | 4
      | 4
      | 4
      | 4
      | 4
      | 4
      | 4
      | 4
      | 4
      | 4
      | 4
      | 4
      | 4
      | 4
      | 4
      | 3
      | 3
      | 3
      | 3
      | 3
      | 3
      | 3
      | 3
      | 3
      | 3
      | 3
      | 2
      | 2
      | 2
      | 2
      | 2
      | 2
      | 2
      | 2
      | 2
      | 2
      | 2
      | 2
      | 2
      | 2
      | 3
      | 3
      | 3
      | 3
      | 3
      | 3
      | 3
      | 3
      | 3
      | 3
      | 3
      | 3
      | 3
      | 3
      | 0
      | 0
      | 0
      | 0
      | 0
      | 0
      | 0
      | 0
      | 0
      | 0
      | 0
      | 0
      | 0
      | 1
      | 1
      | 1
      | 1
      | 1
      | 1
      | 1
      | 2
      | 2
      | 2
      | 2
      | 2
      | 3
      | 3
      | 3
      | 3
      | 3
      | 3
      | 3
      | 3
      | 3
      | 3
      | 3
      | 3
      | 3
      | 3
      | 3
      | 3
      | 3
      | 3
      | 3
      | 3
      | 3
      | 3
      | 3
      | 3
      | 3
      | 3
      | 3
      | 2
      | 2
      | 2
      | 2
      | 2
      | 2
      | 2
      | 2
      | 2
      | 2
      | 2
      | 3
      | 3
      | 3
      | 0
      | 0
      | 0
      | 0
      | 0
      | 0
      | 0
      | 0
      | 0
      | 0
      | 0
      | 0
      | 0
      | 0
      | 0
      | 0
      | 0
      | 0
      | 0
      | 0
      | 0
      | 0
      | 0
      | 0
      | 0
      | 0
      | 0
      | 0
      | 0
      | 0
      | 0
      | 0
      | 0
      | 0
      | 1
      | 1
      | 1
      | 1
      | 1
      | 2
      | 2
      | 2
      | 2
      | 2
      | 2
      | 2
      | 2
      | 2
      | 2
      | 2
      | 2
      | 2
      | 2
      | 2
      | 2
      | 2
      | 2
      | 2
      | 2
      | 2
      | 2
      | 2
      | 2
      | 2
      | 0
      | 0
      | 0
      | 0
      | 0
      | 0
      | 0
      | 0
      | 0
      | 0
      | 0
      | 0
      | 0
      | 0
      | 0
      | 0
      | 0
      | 1
      | 1
      | 1
      | 1
      | 1
      | 1
      | 1
      | 1
      | 1
      | 1
      | 1
      | 1
      | 1
      | 1
      | 1
      | 1
      | 0
      | 0
      | 0
      | 0
      | 0
      | 0
      | 0
      | 0
      | 0
      | 0
      | 0
      | 0
      | 0
      | 0
      | 0
      | 0
      | 0
      | 0
      | 0
      | 0
      | 0
      | 0
      | 0
      | 0
      | 0
      | 0
      | 0
      | 1
      | 1
      | 1
      | 1
      | 1
      | 1
      | 1
      | 0
      | 0
      | 0
      | 0
      | 1
      | 1
      | 1
      | 1
      | 1
      | 1
      | 1
      | 1
      | 0
      | 0
      | 0
      | 0
      | 0
      | 0
      | 0
      | 0
      | 0
      | 0
      | 0
      | 0
      | 0
      | 0
      | 0
      | 0
      | 0
      | 0
      | 0
      | 0
      | 0
      | 0
      | 0
      | 0
      | 0
      | 0
      | 0
      | 0
      | 0
      | 0
      | 0
      | 0
      | 0
      | 0
      | 0
      | 0
      | 0
      | 0
      | 0
      | 0
      | 0
      | 0
      | 0
      | 0
      | 0
      | 0
      | 0
      | 0
      | 0
      | 0
      | 0
      | 0
      | 0
      | 0
      | 0
      | 0
      | 0
      | 0
      | 0
      | 0
      | 0
      | 0
      | 0
      | 0
      | 0
      | 1
      | 1
      | 1
      | 1
      | 1
      | 1
      | 1
      | 1
      | 1
      | 1
      | 1
      | 1
      | 1
      | 1
      | 2
      | 2
      | 2
      | 2
      | 2
      | 2
      | 2
      | 2
      | 2
      | 2
      | 2
      | 2
      | 2
      | 2
      | 1
      | 1
      | 1
      | 1
      | 1
      | 0
      | 0
      | 0
      | 0
      | 0
      | 0
      | 0
      | 0
      | 0
      | 0
      | 0
      | 0
      | 0
      | 0
      | 0
      | 0
      | 0
      | 0
      | 1
      | 1
      | 1
      | 1
      | 1
      | 1
      | 1
      | 1
      | 1
      | 1
      | 1
      | 1
      | 1
      | 1
      | 1
      | 1
      | 1
      | 1
      | 1
      | 1
      | 1
      | 1
      | 1
      | 1
      | 1
      | 1
      | 1
      | 1
      | 1
      | 1
      | 1
      | 1
      | 1
      | 1
      | 1
      | 1
      | 1
      | 1
      | 2
      | 2
      | 2
      | 2
      | 2
      | 2
      | 2
      | 2
      | 2
      | 2
      | 2
      | 2
      | 2
      | 2
      | 2
      | 2
      | 2
      | 2
      | 2
      | 2
      | 2
      | 2
      | 2
      | 0
      | 0
      | 0
      | 0
      | 0
      | 0
      | 0
      | 0
      | 0
      | 0
      | 0
      | 0
      | 0
      | 0
      | 1
      | 1
      | 1
      | 1
      | 1
      | 1
      | 1
      | 1
      | 1
      | 1
      | 1
      | 1
      | 1
      | 1
      | 1
      | 1
      | 0
      | 0
      | 1
      | 1
      | 1
      | 1
      | 1
      | 0
      | 0
      | 1
      | 1
      | 1
      | 1
      | 1
      | 0
      | 0
      | 1
      | 1
      | 1
      | 1
      | 1
      | 1
      | 0
      | 0
      | 1
      | 1
      | 0
      | 0
      | 0
      | 0
      | 0
      | 0
      | 0
      | 0
      | 1
      | 1
      | 1
      | 1
      | 1
      | 1
      | 1
      | 1
      | 1
      | 1
      | 1
      | 2
      | 2
      | 2
      | 2
      | 2
      | 2
      | 2
      | 2
      | 2
      | 2
      | 2
      | 2
      | 2
      | 2
      | 2
      | 2
      | 1
      | 1
      | 1
      | 1
      | 1
      | 1
      | 1
      | 1
      | 1
      | 1
      | 1
      | 2
      | 2
      | 2
      | 2
      | 2
      | 2
      | 2
      | 0
      | 0
      | 0
      | 0
      | 0
      | 1
      | 1
      | 1
      | 1
      | 1
      | 1
      | 1
      | 2
      | 2
      | 2
      | 2
      | 2
      | 2
      | 2
      | 2
      | 2
      | 2
      | 2
      | 2
      | 1
      | 1
      | 1
      | 1
      | 1
      | 2
      | 2
      | 2
      | 2
      | 2
      | 2
      | 2
      | 2
      | 2
      | 2
      | 2
      | 2
      | 2
      | 2
      | 2
      | 2
      | 2
      | 2
      | 2
      | 2
      | 2
      | 2
      | 2
      | 2
      | 2
      | 2
      | 2
      | 0
      | 0
      | 0
      | 0
      | 0
      | 0
      | 0
      | 0
      | 0
      | 0
      | 0
      | 0
      | 0]
  V (km/h) : Outport
  Gear : Outport  Port=2
  wires:
  U Cycle G/1 -> Gear/1
  " U Cycle V"/1 -> V (km/h)/1
  In1/1 -> U Cycle G/1, " U Cycle V"/1
